simulink model "GroundTest"  (R2015a)
settings: configuration reference "GlobalConfig" (kept outside this file)
PreLoadFcn:
  | testModelPreLoadClbck
model workspace (MAT data in the model file):
  MeshNum = Simulink.Parameter
  MeshNum.Value = 20
  MeshNum.DataType = 'auto'
settings Model: Creator=Oleg  LastModifiedBy=Oleg
settings ConfigSetRef: SourceLocation=Base Workspace

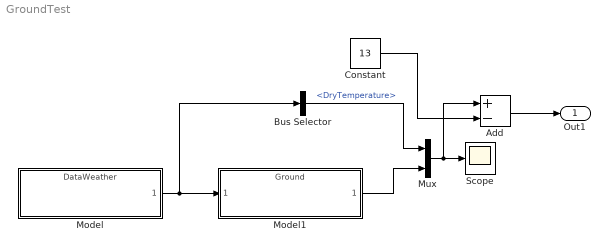
== system GroundTest ==
  Add : Sum  Inputs=+-
  Bus Selector : BusSelector  OutputSignals=DryTemperature
  Constant : Constant  Value=13
  Model : ModelReference  ModelNameDialog=DataWeather.slx  SimulationMode=Normal  ModelReferenceVersion=1.65  CopyOfModelName=DataWeather.slx  DefaultDataLogging=on
  Model1 : ModelReference  ModelNameDialog=Ground.slx  SimulationMode=Normal  ModelReferenceVersion=1.105  CopyOfModelName=Ground.slx  DefaultDataLogging=on
  Mux : Mux  Inputs=2
  Scope : Scope
      settings: YMin=265  YMax=305  MaxDataPoints=1000000
  Out1 : Outport
  wires:
  Model/1 -> Model1/1, Bus Selector/1
  Model1/1 -> Mux/2
  Bus Selector/1 -> Mux/1  "<DryTemperature>"
  Mux/1 -> Add/1, Scope/1
  Add/1 -> Out1/1
  Constant/1 -> Add/2
